simulink model "SIL_test_harness_for_LogicUnderTest"  (R2018b)
settings: Solver=VariableStepAuto  StartTime=0.0  StopTime=10.0  RelTol=1e-3
settings Model: Creator=marwan  LastModifiedBy=marwan
settings DataIOCC: LoadExternalInput=on  OutputSaveName=mdl_out  LoggingToFile=on  LoggingFileName=mdl_out.mat
settings HardwareCC: ProdBitPerPointer=32  ProdBitPerSizeT=32  ProdBitPerPtrDiffT=32  ProdLargestAtomicFloat=None  ProdWordSize=32  ProdHWDeviceType=Atmel->AVR (32-bit)

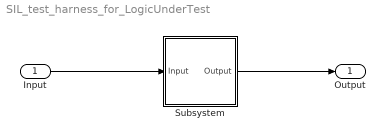
== system SIL_test_harness_for_LogicUnderTest ==
  Input : Inport
  Subsystem : Subsystem  TreatAsAtomicUnit=on
  Output : Outport
  wires:
  Input/1 -> Subsystem/1(Input)
  Subsystem/1(Output) -> Output/1

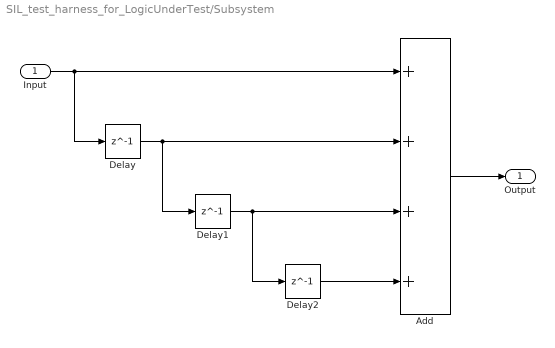
== system SIL_test_harness_for_LogicUnderTest/Subsystem ==
  Input : Inport
  Add : Sum  Inputs=4
  Delay : Delay  DelayLength=1
  Delay1 : Delay  DelayLength=1
  Delay2 : Delay  DelayLength=1
  Output : Outport
  wires:
  Delay/1 -> Delay1/1, Add/2
  Input/1 -> Delay/1, Add/1
  Delay2/1 -> Add/4
  Add/1 -> Output/1
  Delay1/1 -> Delay2/1, Add/3
